simulink model "v2016"  (R2017b)
settings: Solver=VariableStepAuto  StartTime=0.0  StopTime=inf  RelTol=1e-3
undefined symbols (not defined in the file or in its folder): serial
libraries: instrumentlib x3
settings Model: Creator=tomej  LastModifiedBy=tomej

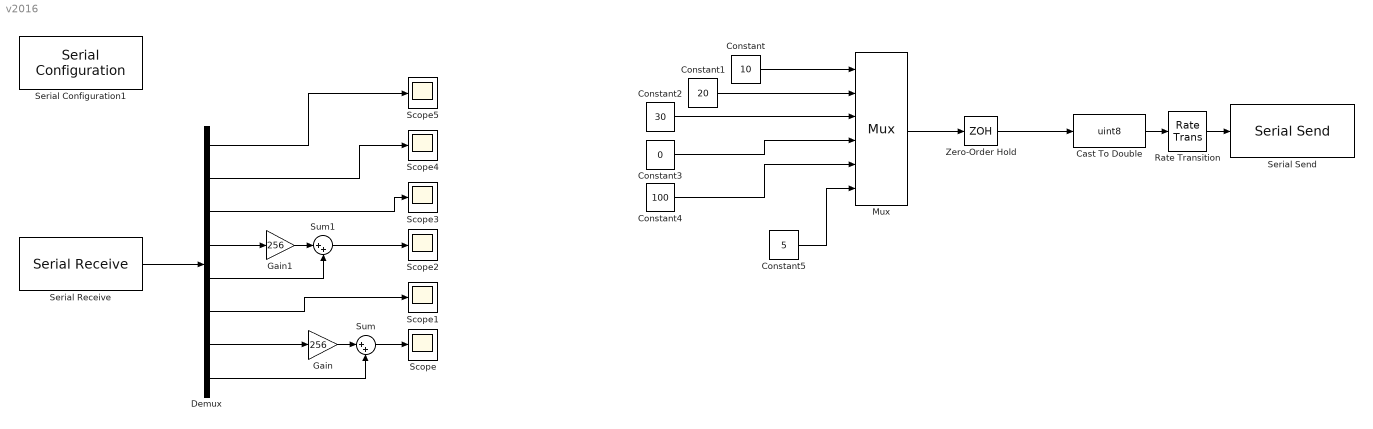
== system v2016 ==
  Cast To Double : DataTypeConversion  OutDataTypeStr=uint8
  Constant : Constant  Value=10
  Constant1 : Constant  Value=20
  Constant2 : Constant  Value=30
  Constant3 : Constant  Value=0
  Constant4 : Constant  Value=100
  Constant5 : Constant  Value=5
  Demux : Demux  Outputs=8
  Gain : Gain  Gain=256
  Gain1 : Gain  Gain=256
  Mux : Mux  Inputs=6
      settings: DisplayOption=signals
  Rate Transition : RateTransition  OutPortSampleTimeOpt=Multiple of input port sample time
  Scope{,1..5} (6 alike) : Scope
  Serial Configuration1 : instrumentlib/Serial Configuration  Priority=-200000  ComPortMenu=<Please select a port...>  ComPort=COM5  ObjConstructor=serial('COM5');  BaudRate=9600  DataBits=8  Parity=none  StopBits=1  FlowControl=none  Timeout=10  ByteOrder=LittleEndian
  Serial Receive : instrumentlib/Serial Receive  ComPortMenu=<Please select a port...>  ComPort=COM5  ObjConstructor=serial('COM5');  Header=efgh  Terminator=<none>  DataSize="[8  1]"  DataType=uint8  EnableBlockingMode=on  ActionDataUnavailable=Output last received value  CustomValue=0  SampleTime=0.01
  Serial Send : instrumentlib/Serial Send  ComPortMenu=<Please select a port...>  ComPort=COM5  ObjConstructor=serial('COM5');  Header=abcd  Terminator=<none>  EnableBlockingMode=on
  Sum : Sum  Inputs=|++
  Sum1 : Sum  Inputs=|++
  Zero-Order Hold : ZeroOrderHold  SampleTime=0.1
  wires:
  Serial Receive/1 -> Demux/1
  Gain/1 -> Sum/1
  Sum/1 -> Scope/1
  Demux/7 -> Gain/1
  Demux/8 -> Sum/2
  Demux/6 -> Scope1/1
  Demux/4 -> Gain1/1
  Gain1/1 -> Sum1/1
  Demux/5 -> Sum1/2
  Sum1/1 -> Scope2/1
  Demux/1 -> Scope5/1
  Demux/2 -> Scope4/1
  Demux/3 -> Scope3/1
  Zero-Order Hold/1 -> Cast To Double/1
  Mux/1 -> Zero-Order Hold/1
  Constant/1 -> Mux/1
  Constant1/1 -> Mux/2
  Constant2/1 -> Mux/3
  Constant3/1 -> Mux/4
  Constant4/1 -> Mux/5
  Constant5/1 -> Mux/6
  Cast To Double/1 -> Rate Transition/1
  Rate Transition/1 -> Serial Send/1
